simulink model "discretezeropole"  (Simulink 7.6)
settings: Solver=FixedStepDiscrete  StartTime=0.0  StopTime=10.0  FixedStep=1  RelTol=1e-3
settings Model: Creator=hnine  LastModifiedBy=hnine
settings OptimizationCC: InitFltsAndDblsToZero=on
settings DebuggingCC: SaveWithParameterizedLinksMsg=none  StrictBusMsg=Warning
settings GRTTargetCC: TargetFcnLib=ansi_tfl_tmw.mat

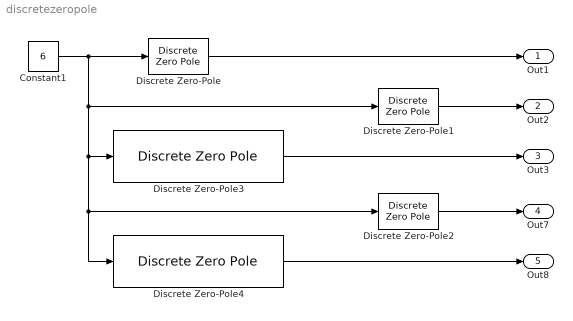
== system discretezeropole ==
  Constant1 : Constant  Value=6  OutDataTypeStr=double
  Discrete Zero-Pole : DiscreteZeroPole  Zeros=[]  Poles=[]  Gain=2
  Discrete Zero-Pole1 : DiscreteZeroPole  Zeros=[]  Poles=[0.05317]  Gain=1
  Discrete Zero-Pole2 : DiscreteZeroPole  Zeros=[-5]  Poles=[-0.5]  Gain=0.2
  Discrete Zero-Pole3 : DiscreteZeroPole  Zeros=[]  Poles=[2.482002 0.332997]  Gain=1
  Discrete Zero-Pole4 : DiscreteZeroPole  Zeros=[-5]  Poles=[2.482002 0.332997]  Gain=0.2
  Out1 : Outport
  Out2 : Outport  Port=2
  Out3 : Outport  Port=3
  Out7 : Outport  Port=4
  Out8 : Outport  Port=5
  wires:
  Constant1/1 -> Discrete Zero-Pole3/1, Discrete Zero-Pole2/1, Discrete Zero-Pole4/1, Discrete Zero-Pole1/1, Discrete Zero-Pole/1
  Discrete Zero-Pole/1 -> Out1/1
  Discrete Zero-Pole1/1 -> Out2/1
  Discrete Zero-Pole3/1 -> Out3/1
  Discrete Zero-Pole2/1 -> Out7/1
  Discrete Zero-Pole4/1 -> Out8/1
